simulink model "design_project_openloop_linear_bk_2"  (R2023b)
settings: Solver=VariableStepAuto  StartTime=0.0  StopTime=500  RelTol=1e-3
settings Model: Creator=qingyu  LastModifiedBy=qingyu

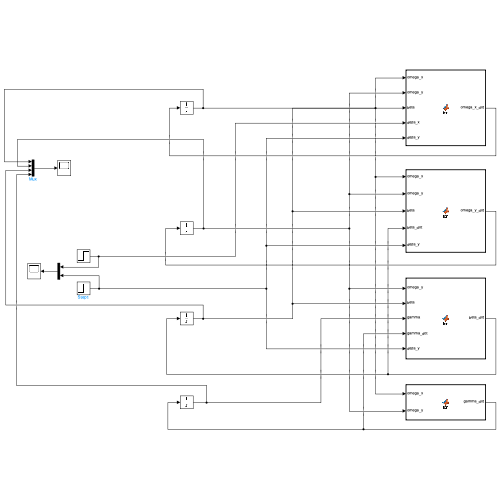
[thumbnail: Simulink's stored preview of the top-level diagram]
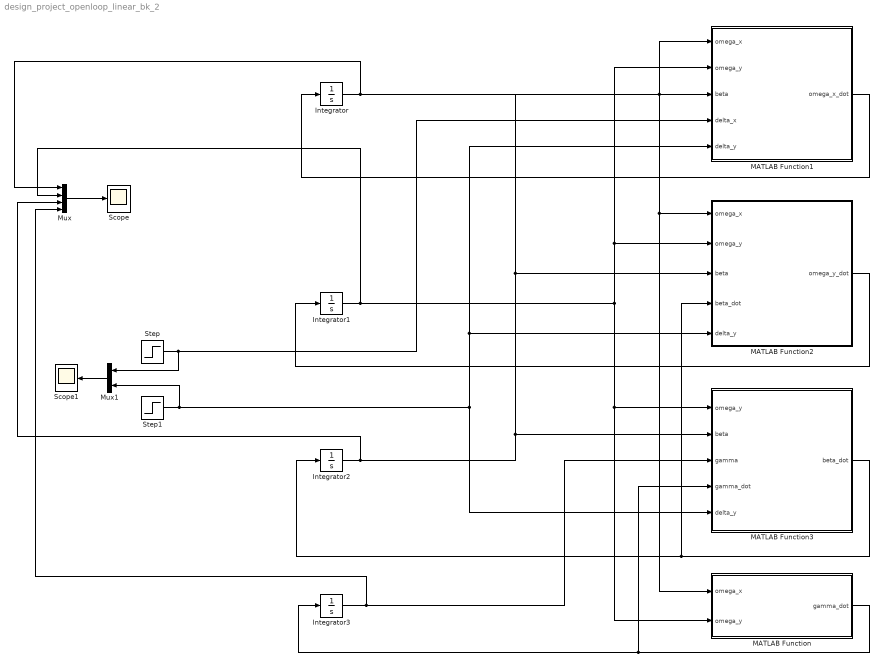
== system design_project_openloop_linear_bk_2 ==
  Integrator : Integrator  InitialCondition=0.1
  Integrator1 : Integrator  InitialCondition=0.1
  Integrator2 : Integrator  InitialCondition=0.05
  Integrator3 : Integrator  InitialCondition=0.05
  MATLAB Function : MATLAB Function  TreatAsAtomicUnit=on
  MATLAB Function1 : MATLAB Function  TreatAsAtomicUnit=on
  MATLAB Function2 : MATLAB Function  TreatAsAtomicUnit=on
  MATLAB Function3 : MATLAB Function  TreatAsAtomicUnit=on
  Mux : Mux
  Mux1 : Mux  Inputs=2
  Scope : Scope
  Scope1 : Scope
  Step : Step  After=0  SampleTime=0
  Step1 : Step  After=0  SampleTime=0
  wires:
  Integrator/1 -> Mux/1, MATLAB Function/1(omega_x), MATLAB Function2/1(omega_x), MATLAB Function1/1(omega_x)
  Integrator1/1 -> Mux/2, MATLAB Function/2(omega_y), MATLAB Function3/1(omega_y), MATLAB Function1/2(omega_y), MATLAB Function2/2(omega_y)
  Integrator2/1 -> Mux/3, MATLAB Function2/3(beta), MATLAB Function1/3(beta), MATLAB Function3/2(beta)
  Integrator3/1 -> Mux/4, MATLAB Function3/3(gamma)
  Step/1 -> Mux1/1, MATLAB Function1/4(delta_x)
  Step1/1 -> Mux1/2, MATLAB Function1/5(delta_y), MATLAB Function2/5(delta_y), MATLAB Function3/5(delta_y)
  MATLAB Function1/1(omega_x_dot) -> Integrator/1
  MATLAB Function2/1(omega_y_dot) -> Integrator1/1
  MATLAB Function3/1(beta_dot) -> Integrator2/1, MATLAB Function2/4(beta_dot)
  MATLAB Function/1(gamma_dot) -> Integrator3/1, MATLAB Function3/4(gamma_dot)
  Mux/1 -> Scope/1
  Mux1/1 -> Scope1/1

== matlab function design_project_openloop_linear_bk_2/MATLAB Function1 ==
  data: omega_x input; omega_x_dot output; omega_y input; beta input; delta_x input; delta_y input

function omega_x_dot = fcn(omega_x, omega_y, beta, delta_x, delta_y)

J_x             =  2.601;
M_x_omega_x     = -4.8379;
M_x_omega_y     = -1.7167;
M_x_beta        = -22.8888;
M_x_delta_x     = -2.5490;
M_x_delta_y     = -2.0289;

omega_x_dot = 0;
omega_x_dot = omega_x_dot + M_x_omega_x/J_x*omega_x;
omega_x_dot = omega_x_dot + M_x_omega_y/J_x*omega_y;
omega_x_dot = omega_x_dot + M_x_beta/J_x*beta;
omega_x_dot = omega_x_dot + M_x_delta_x/J_x*delta_x;
omega_x_dot = omega_x_dot + M_x_delta_y/J_x*delta_y;

== matlab function design_project_openloop_linear_bk_2/MATLAB Function ==
  data: omega_x input; gamma_dot output; omega_y input
function gamma_dot = fcn(omega_x,omega_y)

vartheta = 0.1930;

gamma_dot = 0;
gamma_dot = gamma_dot + omega_x;
gamma_dot = gamma_dot - tand(vartheta)*omega_y;

== matlab function design_project_openloop_linear_bk_2/MATLAB Function2 ==
  data: omega_x input; omega_y_dot output; omega_y input; beta input; beta_dot input; delta_y input
function omega_y_dot = fcn(omega_x,omega_y,beta,beta_dot,delta_y)

J_y             =  751.8960;
M_y_omega_x     = -15.0379;
M_y_omega_y     = -150.3792;
M_y_beta        = -2255.6880;
M_y_beta_dot    =  0;
M_y_delta_y     = -676.7064;

omega_y_dot = 0;
omega_y_dot = omega_y_dot + M_y_omega_x/J_y*omega_x;
omega_y_dot = omega_y_dot + M_y_omega_y/J_y*omega_y;
omega_y_dot = omega_y_dot + M_y_beta/J_y*beta;
omega_y_dot = omega_y_dot + M_y_beta_dot/J_y*beta_dot;
omega_y_dot = omega_y_dot + M_y_delta_y/J_y*delta_y;

== matlab function design_project_openloop_linear_bk_2/MATLAB Function3 ==
  data: omega_y input; beta input; gamma input; beta_dot output; gamma_dot input; delta_y input
function beta_dot = fcn(omega_y, beta, gamma, gamma_dot, delta_y)

g               =  9.81;
v               =  350.3552;
m               =  320;
P               =  20000;
alpha           =  0.2618;
theta           = -0.0688;
vartheta        =  0.1930;
Z_delta_y       = -2018.0457;
Z_beta          =  13273.1810;

beta_dot = 0;
beta_dot = beta_dot + cosd(theta)/cosd(vartheta)*omega_y;
beta_dot = beta_dot - (P-Z_beta)/(m*v)*beta;
beta_dot = beta_dot + (g/v)*sind(theta)*beta;
beta_dot = beta_dot + (g/v)*cosd(vartheta)*gamma;
beta_dot = beta_dot + alpha*gamma_dot;
beta_dot = beta_dot + Z_delta_y/(m*v)*delta_y;
